simulink model "GP"  (R2013a)
settings: Solver=ode45  StartTime=0.0  StopTime=5  FixedStep=0.1  RelTol=0.1
libraries: simulink_extras x6, aerolibnav x2, aerolibutil x1, dspmathops x1
settings Model: Creator=Nour  LastModifiedBy=Ibrahim_B92

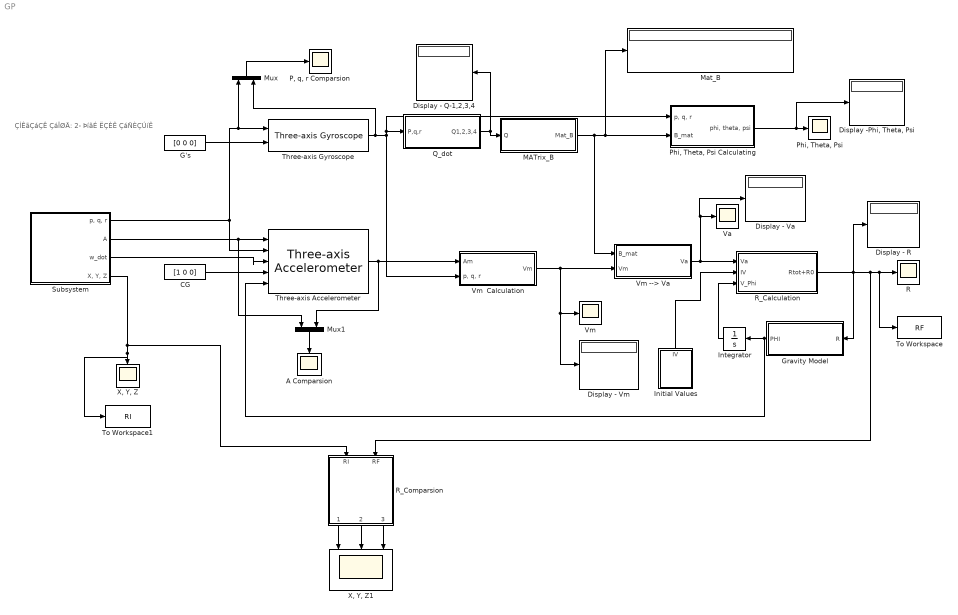
== system GP ==
  note: ÇÍÊãÇáÇÊ ÇáÎØÃ:
      | 2- ÞíãÉ ËÇÈÊ ÇáÑÈÇÚíÊ
  A Comparsion : Scope
      settings: TimeRange=3  YMin=-30  YMax=10  SaveName=ScopeData9
  CG : Constant  Value=[1 0 0]
  Display - Q-1,2,3,4 : Display
  Display - R : Display
  Display - Va : Display
  Display - Vm : Display
  "Display -Phi, Theta, Psi" : Display
  G's : Constant  Value=[0 0 0]
  "Gravity Model " : Subsystem
  "Initial Values " : Subsystem
  Integrator : Integrator
  MATrix_B : Subsystem
  Mat_B : Display
  Mux : Mux  Inputs=2
  Mux1 : Mux  Inputs=2
  "P, q, r Comparsion" : Scope
      settings: YMin=-0.6  YMax=0.8  SaveName=ScopeData8
  "Phi, Theta, Psi" : Scope
  "Phi, Theta, Psi Calculating" : Subsystem
  Q_dot : Subsystem
  R : Scope
      settings: YMin=-3.5e+09  YMax=3.5e+09  SaveName=ScopeData2
  R_Calculation : Subsystem
  R_Comparsion : Subsystem
  Subsystem : Subsystem
  Three-axis Accelerometer : aerolibnav/Three-axis Accelerometer  units=Metric (MKS)  acc=[1 0 0]  gtype=on  dtype_a=on  w_a=190  z_a=0.707  a_sf_cc=[1 0 0; 0 1 0; 0 0 1]  a_bias=[0 0 0]  a_rand=on  a_seeds=[23093 23094 23095]  a_pow=[0.0001 0.0001 0.0001]  a_sat="[-inf  -inf  -inf  inf inf inf]"  a_Ts=0
  Three-axis Gyroscope : aerolibnav/Three-axis Gyroscope  dtype_g=on  w_g=190  z_g=0.707  g_sf_cc=[1 0 0; 0 1 0; 0 0 1]  g_bias=[0 0 0]  g_sen=[0 0 0]  g_rand=on  g_seeds=[23093 23094 23095]  g_pow=[0.00005 0.00005 0.00005]  g_sat="[-inf  -inf  -inf  inf inf inf]"  g_Ts=0
  To Workspace : ToWorkspace  VariableName=RF  SampleTime=-1
      settings: Decimation=3
  To Workspace1 : ToWorkspace  VariableName=RI  SampleTime=-1
      settings: Decimation=3
  Va : Scope
      settings: SaveName=ScopeData4
  Vm : Scope
      settings: SaveName=ScopeData3
  Vm  Calculation : Subsystem
  Vm --> Va : Subsystem
  "X, Y, Z" : Scope
      settings: TimeRange=3  YMin=-30  YMax=10
  "X, Y, Z1" : Scope  NumInputPorts=3
      settings: TimeRange=5  YMin=-275~-75~0  YMax=25~100~150  SaveName=ScopeData5
  wires:
  Q_dot/1(Q1,2,3,4) -> MATrix_B/1(Q), Display - Q-1,2,3,4/1
  MATrix_B/1(Mat_B) -> Vm --> Va/1(B_mat), "Phi, Theta, Psi Calculating"/2(B_mat), Mat_B/1
  Vm  Calculation/1(Vm) -> Display - Vm/1, Vm/1, Vm --> Va/2(Vm)
  "Initial Values "/1(IV) -> R_Calculation/2(IV)
  Vm --> Va/1(Va) -> Va/1, Display - Va/1, R_Calculation/1(Va)
  R_Calculation/1(Rtot+R0) -> Display - R/1, R_Comparsion/2(RF), To Workspace/1, R/1, "Gravity Model "/1(R)
  Integrator/1 -> R_Calculation/3(V_Phi)
  Subsystem/1("p, q, r") -> Three-axis Gyroscope/1, Mux/1, Three-axis Accelerometer/2
  Subsystem/3(w_dot) -> Three-axis Accelerometer/3
  CG/1 -> Three-axis Accelerometer/4
  "Gravity Model "/1(PHI) -> Integrator/1, Three-axis Accelerometer/5
  G's/1 -> Three-axis Gyroscope/2
  "Phi, Theta, Psi Calculating"/1("phi, theta, psi") -> "Display -Phi, Theta, Psi"/1, "Phi, Theta, Psi"/1
  Three-axis Gyroscope/1 -> Mux/2, Q_dot/1(P,q,r), "Phi, Theta, Psi Calculating"/1("p, q, r"), Vm  Calculation/2("p, q, r")
  Mux/1 -> "P, q, r Comparsion"/1
  Mux1/1 -> A Comparsion/1
  Subsystem/2(A) -> Mux1/1, Three-axis Accelerometer/1
  Three-axis Accelerometer/1 -> Mux1/2, Vm  Calculation/1(Am)
  Subsystem/4("X, Y, Z") -> R_Comparsion/1(RI), To Workspace1/1, "X, Y, Z"/1
  R_Comparsion/1(X_Comarsion) -> "X, Y, Z1"/1
  R_Comparsion/2(Y_Comarsion1) -> "X, Y, Z1"/2
  R_Comparsion/3(Z_Comarsion2) -> "X, Y, Z1"/3

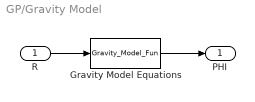
== system GP/Gravity Model  ==
  R : Inport
  Gravity Model Equations : MATLABFcn  MATLABFcn=Gravity_Model_Fun  OutputDimensions=3
  PHI : Outport
  wires:
  R/1 -> Gravity Model Equations/1
  Gravity Model Equations/1 -> PHI/1

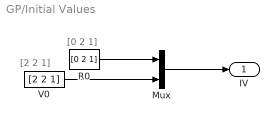
== system GP/Initial Values  ==
  note: [2 2 1]
  note: [0 2 1]
  Mux : Mux  Inputs=2
  R0 : Constant  Value=[0 2 1]
  V0 : Constant  Value=[2 2 1]
  IV : Outport
  wires:
  R0/1 -> Mux/1
  V0/1 -> Mux/2
  Mux/1 -> IV/1

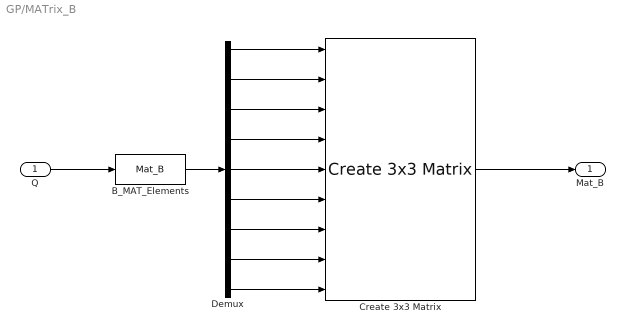
== system GP/MATrix_B ==
  Q : Inport
  B_MAT_Elements : MATLABFcn  MATLABFcn=Mat_B  OutputDimensions=9
  Create 3x3 Matrix : aerolibutil/Create 3x3 Matrix
  Demux : Demux  Outputs=9
  Mat_B : Outport
  wires:
  Q/1 -> B_MAT_Elements/1
  B_MAT_Elements/1 -> Demux/1
  Demux/1 -> Create 3x3 Matrix/1
  Demux/2 -> Create 3x3 Matrix/2
  Demux/3 -> Create 3x3 Matrix/3
  Demux/4 -> Create 3x3 Matrix/4
  Demux/5 -> Create 3x3 Matrix/5
  Demux/6 -> Create 3x3 Matrix/6
  Demux/7 -> Create 3x3 Matrix/7
  Demux/8 -> Create 3x3 Matrix/8
  Demux/9 -> Create 3x3 Matrix/9
  Create 3x3 Matrix/1 -> Mat_B/1

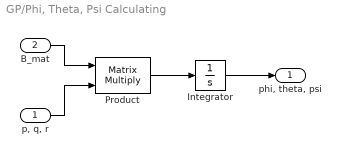
== system GP/Phi, Theta, Psi Calculating ==
  "p, q, r" : Inport
  B_mat : Inport  Port=2
  Integrator : Integrator
  Product : Product  Multiplication=Matrix(*)
  "phi, theta, psi" : Outport
  wires:
  "p, q, r"/1 -> Product/2
  B_mat/1 -> Product/1
  Product/1 -> Integrator/1
  Integrator/1 -> "phi, theta, psi"/1

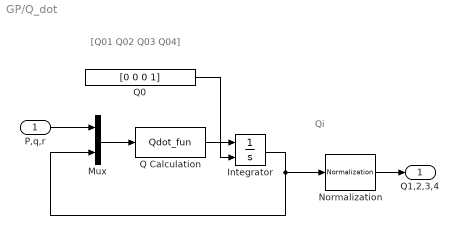
== system GP/Q_dot ==
  note: [Q01 Q02 Q03 Q04]
  note: Qi
  P,q,r : Inport
  Integrator : Integrator  InitialConditionSource=external
  Mux : Mux  Inputs=2
  Normalization : dspmathops/Normalization  NormType=2-norm  Bias=1e-10  NormOver=Each row  ColComp=on  Dimension=4  outputDataTypeStr=Inherit: Same as product output  outputLastDataTypeStr=Inherit: Same as product output  outputMin=[]  outputMax=[]  accumDataTypeStr=Inherit: Same as product output  accumLastDataTypeStr=Inherit: Same as product output  roundingMode=Floor  overflowMode=off
  Q Calculation : MATLABFcn  MATLABFcn=Qdot_fun  OutputDimensions=4
  Q0 : Constant  Value=[0 0 0 1]
  Q1,2,3,4 : Outport
  wires:
  P,q,r/1 -> Mux/1
  Q Calculation/1 -> Integrator/1
  Mux/1 -> Q Calculation/1
  Normalization/1 -> Q1,2,3,4/1
  Integrator/1 -> Normalization/1, Mux/2
  Q0/1 -> Integrator/2

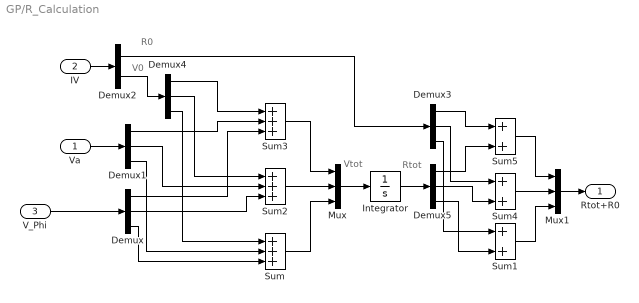
== system GP/R_Calculation ==
  note: Rtot
  note: Vtot
  note: V0
  note: R0
  Va : Inport
  IV : Inport  Port=2
  V_Phi : Inport  Port=3
  Demux{,1,3..5} (5 alike) : Demux  Outputs=3
  Demux2 : Demux  Outputs=2
  Integrator : Integrator  InitialCondition=[0 0 0]
  Mux : Mux  Inputs=3
  Mux1 : Mux  Inputs=3
  Sum : Sum  Inputs=+++
  Sum1 : Sum
  Sum2 : Sum  Inputs=+++
  Sum3 : Sum  Inputs=+++
  Sum4 : Sum
  Sum5 : Sum
  Rtot+R0 : Outport
  wires:
  Va/1 -> Demux1/1
  Demux2/1 -> Demux3/1
  Demux2/2 -> Demux4/1
  IV/1 -> Demux2/1
  Demux4/1 -> Sum3/1
  Demux1/1 -> Sum3/2
  Demux/1 -> Sum3/3
  Demux4/2 -> Sum2/1
  Demux1/2 -> Sum2/2
  Demux/2 -> Sum2/3
  Demux4/3 -> Sum/1
  Demux1/3 -> Sum/2
  Demux/3 -> Sum/3
  Sum3/1 -> Mux/1
  Sum2/1 -> Mux/2
  Sum/1 -> Mux/3
  Mux/1 -> Integrator/1
  Integrator/1 -> Demux5/1
  Demux3/1 -> Sum5/1
  Demux5/1 -> Sum5/2
  Demux3/2 -> Sum4/1
  Demux5/2 -> Sum4/2
  Demux3/3 -> Sum1/1
  Demux5/3 -> Sum1/2
  Sum4/1 -> Mux1/2
  Sum5/1 -> Mux1/1
  Sum1/1 -> Mux1/3
  Mux1/1 -> Rtot+R0/1
  V_Phi/1 -> Demux/1

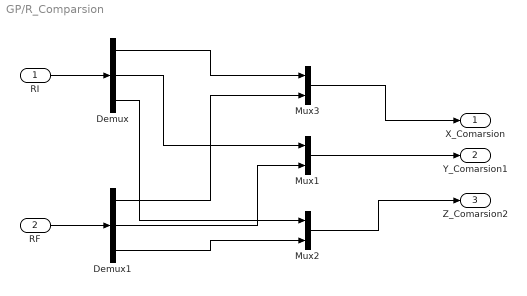
== system GP/R_Comparsion ==
  RI : Inport
  RF : Inport  Port=2
  Demux : Demux  Outputs=3
  Demux1 : Demux  Outputs=3
  Mux1 : Mux  Inputs=2
  Mux2 : Mux  Inputs=2
  Mux3 : Mux  Inputs=2
  X_Comarsion : Outport
  Y_Comarsion1 : Outport  Port=2
  Z_Comarsion2 : Outport  Port=3
  wires:
  RI/1 -> Demux/1
  RF/1 -> Demux1/1
  Demux/1 -> Mux3/1
  Demux1/1 -> Mux3/2
  Demux/2 -> Mux1/1
  Demux1/2 -> Mux1/2
  Demux/3 -> Mux2/1
  Demux1/3 -> Mux2/2
  Mux3/1 -> X_Comarsion/1
  Mux1/1 -> Y_Comarsion1/1
  Mux2/1 -> Z_Comarsion2/1

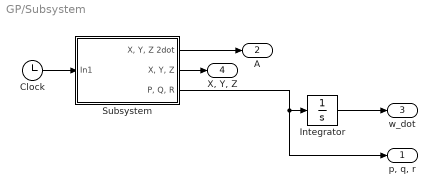
== system GP/Subsystem ==
  Clock : Clock
  Integrator : Integrator
  Subsystem : Subsystem
  "p, q, r" : Outport
  A : Outport  Port=2
  w_dot : Outport  Port=3
  "X, Y, Z" : Outport  Port=4
  wires:
  Clock/1 -> Subsystem/1(In1)
  Subsystem/3("P, Q, R") -> Integrator/1, "p, q, r"/1
  Integrator/1 -> w_dot/1
  Subsystem/1("X, Y, Z 2dot") -> A/1
  Subsystem/2("X, Y, Z") -> "X, Y, Z"/1

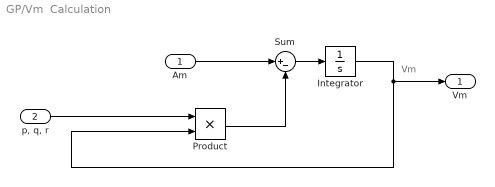
== system GP/Vm  Calculation ==
  note: Vm
  Am : Inport
  "p, q, r" : Inport  Port=2
  Integrator : Integrator
  Product : Product
  Sum : Sum  Inputs=|+-
  Vm : Outport
  wires:
  Am/1 -> Sum/1
  "p, q, r"/1 -> Product/1
  Product/1 -> Sum/2
  Integrator/1 -> Product/2, Vm/1
  Sum/1 -> Integrator/1

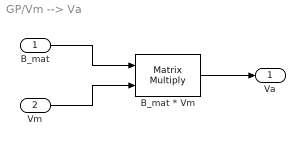
== system GP/Vm --> Va ==
  B_mat : Inport
  Vm : Inport  Port=2
  B_mat * Vm : Product  Multiplication=Matrix(*)
  Va : Outport
  wires:
  B_mat/1 -> B_mat * Vm/1
  Vm/1 -> B_mat * Vm/2
  B_mat * Vm/1 -> Va/1

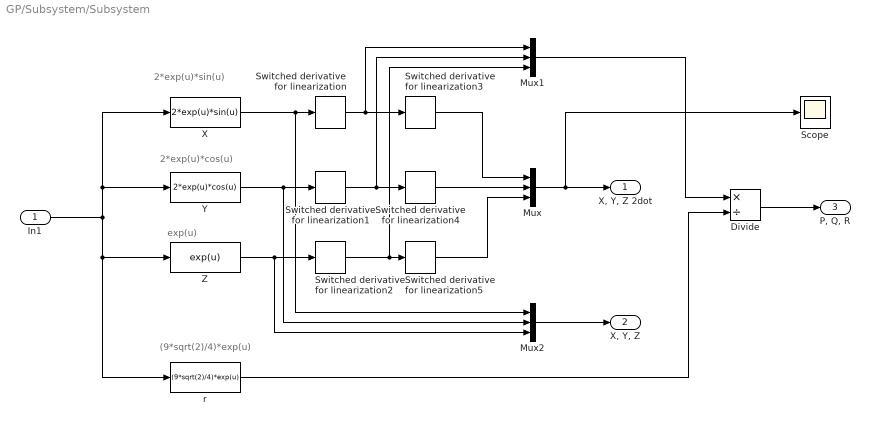
== system GP/Subsystem/Subsystem ==
  note: (9*sqrt(2)/4)*exp(u)
  note: exp(u)
  note: 2*exp(u)*cos(u)
  note: 2*exp(u)*sin(u)
  In1 : Inport
  Divide : Product  Inputs=*/
  Mux : Mux  Inputs=3
  Mux1 : Mux  Inputs=3
  Mux2 : Mux  Inputs=3
  Scope : Scope
      settings: YMin=-50000  YMax=800000  SaveName=ScopeData6
  Switched derivative for linearization{,1..5} (6 alike) : simulink_extras/Linearization/Switched derivative for linearization  switchVal=1  derivConst=1
  X : MATLABFcn  MATLABFcn=2*exp(u)*sin(u)
  Y : MATLABFcn  MATLABFcn=2*exp(u)*cos(u)
  Z : MATLABFcn  MATLABFcn=exp(u)
  r : MATLABFcn  MATLABFcn=(9*sqrt(2)/4)*exp(u)
  "X, Y, Z 2dot" : Outport
  "X, Y, Z" : Outport  Port=2
  "P, Q, R" : Outport  Port=3
  wires:
  In1/1 -> X/1, Y/1, Z/1, r/1
  X/1 -> Switched derivative for linearization/1, Mux2/1
  Y/1 -> Switched derivative for linearization1/1, Mux2/2
  Z/1 -> Switched derivative for linearization2/1, Mux2/3
  Switched derivative for linearization/1 -> Switched derivative for linearization3/1, Mux1/1
  Switched derivative for linearization1/1 -> Switched derivative for linearization4/1, Mux1/2
  Switched derivative for linearization2/1 -> Switched derivative for linearization5/1, Mux1/3
  Mux1/1 -> Divide/1
  Mux/1 -> Scope/1, "X, Y, Z 2dot"/1
  Switched derivative for linearization3/1 -> Mux/1
  Switched derivative for linearization4/1 -> Mux/2
  Switched derivative for linearization5/1 -> Mux/3
  Mux2/1 -> "X, Y, Z"/1
  r/1 -> Divide/2
  Divide/1 -> "P, Q, R"/1
